simulink model "test"  (R2024b)
settings: Solver=ode4  StartTime=0.0  StopTime=10000  FixedStep=0.01  RelTol=1e-3
values from neighbouring files (symbols this model uses):
  db = 0*[-100 100]    [test_workspace.m]
  dwell_param = [Uon; Uoff; min_on; min_off]    [test_workspace.m]
  Fmax_rcs = 500    [test_workspace.m]
  I = 1e5*diag([1.8382, 1.8626, 1.0379])    [test_workspace.m]
  ka = 0.2*kr    [test_workspace.m]
  km = 4    [test_workspace.m]
  kr = [0.5 0.5 0.8]'    [test_workspace.m]
  larm = 2*[4; 4; 4]    [test_workspace.m]
  min_on = 0.03    [test_workspace.m]
  tau = 1    [test_workspace.m]
  Uoff = 0.1    [test_workspace.m]
  Uon = 0.4    [test_workspace.m]
libraries: simulink x1
settings Model: NumberOfSteps=5000  Creator=gabri  LastModifiedBy=gabri

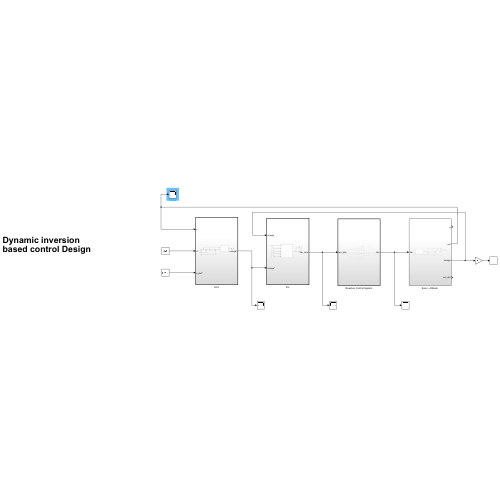
[thumbnail: Simulink's stored preview of the top-level diagram]
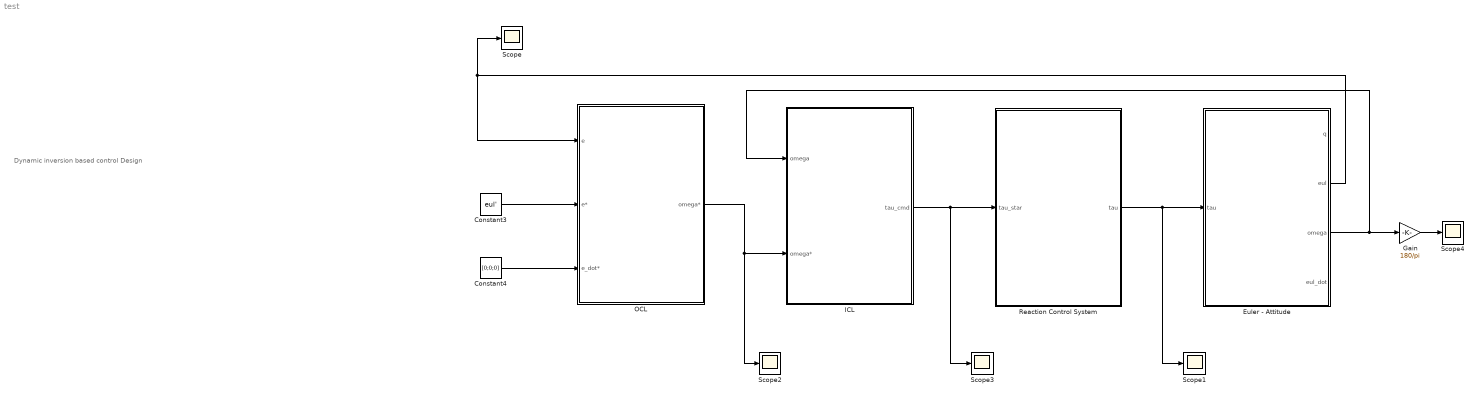
== system test ==
  note: Dynamic inversion based control Design
  Constant3 : Constant  Value=eul'
  Constant4 : Constant  Value=[0;0;0]
  "Euler - Attitude " : Subsystem
  Gain : Gain  Gain=180/pi
  ICL : Subsystem  TreatAsAtomicUnit=on
  OCL : Subsystem  TreatAsAtomicUnit=on
  Reaction Control System : Subsystem  TreatAsAtomicUnit=on
  Scope{,1..4} (5 alike) : Scope
  wires:
  Reaction Control System/1(tau) -> Scope1/1, "Euler - Attitude "/1(tau)
  "Euler - Attitude "/2(eul) -> OCL/1(e), Scope/1
  "Euler - Attitude "/3(omega) -> Gain/1, ICL/1(omega)
  OCL/1(omega*) -> ICL/2(omega*), Scope2/1
  ICL/1(tau_cmd) -> Scope3/1, Reaction Control System/1(tau_star)
  Constant3/1 -> OCL/2(e*)
  Constant4/1 -> OCL/3(e_dot*)
  Gain/1 -> Scope4/1

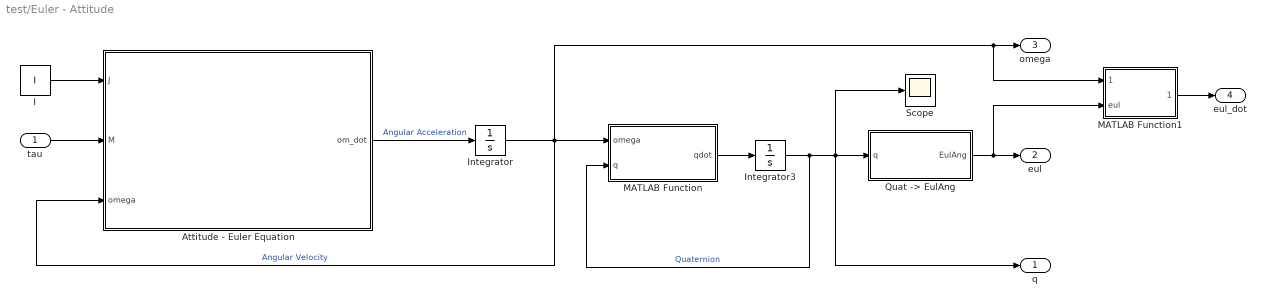
== system test/Euler - Attitude  ==
  tau : Inport
  Attitude - Euler Equation : MATLAB Function  TreatAsAtomicUnit=on
  I : Constant  Value=I
  Integrator : Integrator  InitialCondition=[0; 0; 0]
  Integrator3 : Integrator  InitialCondition=[1; 0; 0; 0]
  MATLAB Function : MATLAB Function  TreatAsAtomicUnit=on
  MATLAB Function1 : MATLAB Function  TreatAsAtomicUnit=on
  "Quat -> EulAng" : MATLAB Function  TreatAsAtomicUnit=on
  Scope : Scope
  q : Outport
  eul : Outport  Port=2
  omega : Outport  Port=3
  eul_dot : Outport  Port=4
  wires:
  Attitude - Euler Equation/1(om_dot) -> Integrator/1  "Angular Acceleration"
  tau/1 -> Attitude - Euler Equation/2(M)
  MATLAB Function/1(qdot) -> Integrator3/1
  Integrator/1 -> MATLAB Function1/1(omega), omega/1, MATLAB Function/1(omega), Attitude - Euler Equation/3(omega)  "Angular Velocity"
  Integrator3/1 -> q/1, "Quat -> EulAng"/1(q), Scope/1, MATLAB Function/2(q)  "Quaternion"
  I/1 -> Attitude - Euler Equation/1(J)
  "Quat -> EulAng"/1(EulAng) -> eul/1, MATLAB Function1/2(eul)
  MATLAB Function1/1(eul_dot) -> eul_dot/1

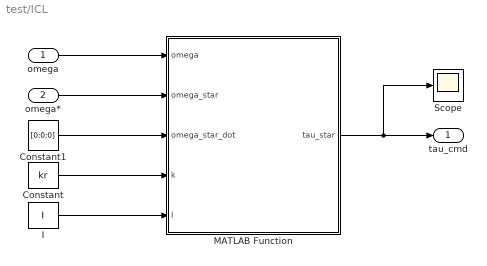
== system test/ICL ==
  omega : Inport
  omega* : Inport  Port=2
  Constant : Constant  Value=kr
  Constant1 : Constant  Value=[0;0;0]
  I : Constant  Value=I
  MATLAB Function : MATLAB Function  TreatAsAtomicUnit=on
  Scope : Scope
  tau_cmd : Outport
  wires:
  omega/1 -> MATLAB Function/1(omega)
  MATLAB Function/1(tau_star) -> Scope/1, tau_cmd/1
  omega*/1 -> MATLAB Function/2(omega_star)
  Constant/1 -> MATLAB Function/4(k)
  I/1 -> MATLAB Function/5(I)
  Constant1/1 -> MATLAB Function/3(omega_star_dot)

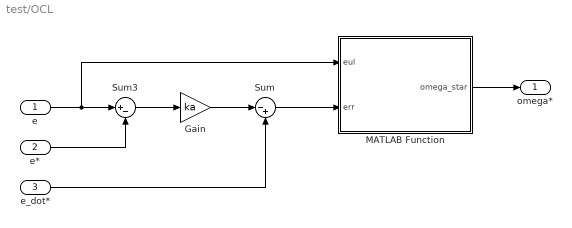
== system test/OCL ==
  e : Inport
  e* : Inport  Port=2
  e_dot* : Inport  Port=3
  Gain : Gain  Gain=ka
  MATLAB Function : MATLAB Function  TreatAsAtomicUnit=on
  Sum : Sum  Inputs=|-+
  Sum3 : Sum  Inputs=|+-
  omega* : Outport
  wires:
  e/1 -> MATLAB Function/1(eul), Sum3/1
  e*/1 -> Sum3/2
  Sum3/1 -> Gain/1
  MATLAB Function/1(omega_star) -> omega*/1
  e_dot*/1 -> Sum/2
  Gain/1 -> Sum/1
  Sum/1 -> MATLAB Function/2(err)

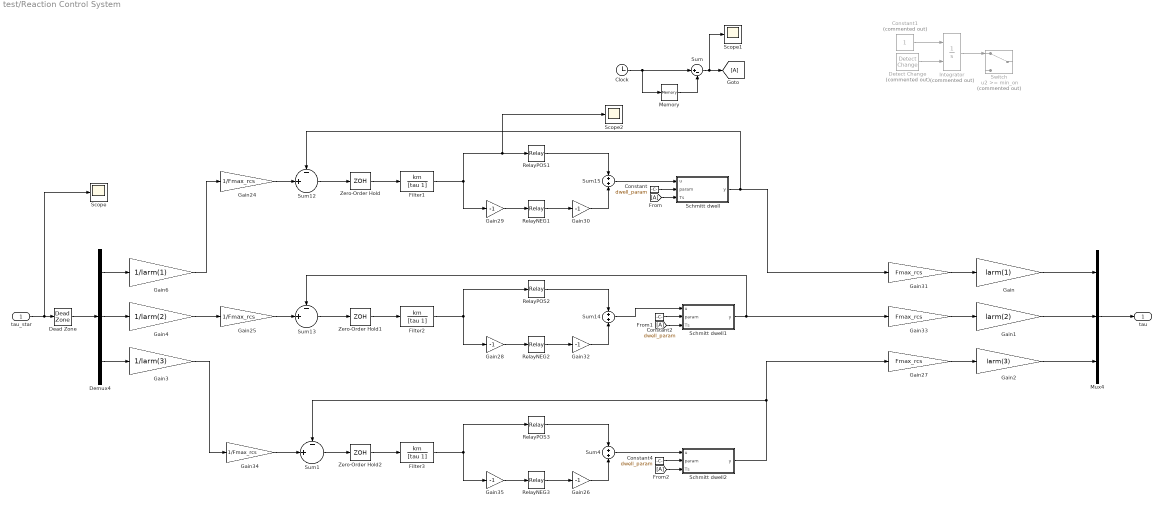
== system test/Reaction Control System ==
  tau_star : Inport
  Clock : Clock
  Constant : Constant  Value=dwell_param
  Constant1 : Constant  Commented=on
  Constant2 : Constant  Value=dwell_param
  Constant4 : Constant  Value=dwell_param
  Dead Zone : DeadZone  LowerValue=db(1)  UpperValue=db(2)
  Demux4 : Demux  Outputs=3
  Detect Change : simulink/Logic and Bit Operations/Detect Change  Commented=on  vinit=0  OutDataTypeStr=boolean
  Filter1 : TransferFcn  Numerator=km  Denominator=[tau 1]
  Filter2 : TransferFcn  Numerator=km  Denominator=[tau 1]
  Filter3 : TransferFcn  Numerator=km  Denominator=[tau 1]
  From : From
  From1 : From
  From2 : From
  Gain : Gain  Gain=larm(1)
  Gain1 : Gain  Gain=larm(2)
  Gain2 : Gain  Gain=larm(3)
  Gain24 : Gain  Gain=1/Fmax_rcs
  Gain25 : Gain  Gain=1/Fmax_rcs
  Gain{26,28..30,32,35} (6 alike) : Gain  Gain=-1
  Gain27 : Gain  Gain=Fmax_rcs
  Gain3 : Gain  Gain=1/larm(3)
  Gain31 : Gain  Gain=Fmax_rcs
  Gain33 : Gain  Gain=Fmax_rcs
  Gain34 : Gain  Gain=1/Fmax_rcs
  Gain4 : Gain  Gain=1/larm(2)
  Gain6 : Gain  Gain=1/larm(1)
  Goto : Goto
  Integrator : Integrator  Commented=on  ExternalReset=level
  Memory : Memory
  Mux4 : Mux  Inputs=3
  RelayNEG1 : Relay  OnSwitchValue=0.45  OffSwitchValue=0.15  ZeroCross=off  SampleTime=0.01
  RelayNEG2 : Relay  OnSwitchValue=Uon  OffSwitchValue=Uoff  ZeroCross=off  SampleTime=0.01
  RelayNEG3 : Relay  OnSwitchValue=0.45  OffSwitchValue=0.15  ZeroCross=off  SampleTime=0.01
  RelayPOS1 : Relay  OnSwitchValue=Uon  OffSwitchValue=Uoff  ZeroCross=off  SampleTime=0.01
  RelayPOS2 : Relay  OnSwitchValue=Uon  OffSwitchValue=Uoff  ZeroCross=off  SampleTime=0.01
  RelayPOS3 : Relay  OnSwitchValue=Uon  OffSwitchValue=Uoff  ZeroCross=off  SampleTime=0.01
  Schmitt dwell : MATLAB Function  TreatAsAtomicUnit=on
  Schmitt dwell1 : MATLAB Function  TreatAsAtomicUnit=on
  Schmitt dwell2 : MATLAB Function  TreatAsAtomicUnit=on
  Scope : Scope
  Scope1 : Scope
  Scope2 : Scope
  Sum : Sum  Inputs=|+-
  Sum1 : Sum  Inputs=-||+|||
  Sum12 : Sum  Inputs=-||+|||
  Sum13 : Sum  Inputs=-||+|||
  Sum14 : Sum  Inputs=+|+
  Sum15 : Sum  Inputs=+|+
  Sum4 : Sum  Inputs=+|+
  Switch : Switch  Commented=on  Threshold=min_on  SaturateOnIntegerOverflow=off  InputSameDT=off
  Zero-Order Hold : ZeroOrderHold  SampleTime=0.01
  Zero-Order Hold1 : ZeroOrderHold  SampleTime=0.01
  Zero-Order Hold2 : ZeroOrderHold  SampleTime=0.01
  tau : Outport
  wires:
  RelayNEG2/1 -> Gain32/1
  RelayNEG3/1 -> Gain26/1
  RelayPOS2/1 -> Sum14/1
  Gain27/1 -> Gain2/1
  Sum4/1 -> Schmitt dwell2/1(u)
  Gain24/1 -> Sum12/2
  Gain30/1 -> Sum15/2
  Filter3/1 -> Gain35/1, RelayPOS3/1
  Gain26/1 -> Sum4/2
  Sum1/1 -> Zero-Order Hold2/1
  Filter2/1 -> Gain28/1, RelayPOS2/1
  RelayPOS3/1 -> Sum4/1
  Demux4/3 -> Gain3/1
  RelayNEG1/1 -> Gain30/1
  Gain28/1 -> RelayNEG2/1
  Demux4/1 -> Gain6/1
  Gain32/1 -> Sum14/2
  Gain31/1 -> Gain/1
  Sum13/1 -> Zero-Order Hold1/1
  Demux4/2 -> Gain4/1
  Sum14/1 -> Schmitt dwell1/1(u)
  Gain33/1 -> Gain1/1
  Gain35/1 -> RelayNEG3/1
  Gain29/1 -> RelayNEG1/1
  Sum12/1 -> Zero-Order Hold/1
  Gain/1 -> Mux4/1
  Gain1/1 -> Mux4/2
  Gain2/1 -> Mux4/3
  tau_star/1 -> Scope/1, Dead Zone/1
  Mux4/1 -> tau/1
  Gain4/1 -> Gain25/1
  Gain3/1 -> Gain34/1
  Integrator/1 -> Switch/1
  Constant1/1 -> Integrator/1
  Detect Change/1 -> Integrator/2
  Sum15/1 -> Schmitt dwell/1(u)
  Filter1/1 -> Scope2/1, RelayPOS1/1, Gain29/1
  RelayPOS1/1 -> Sum15/1
  From/1 -> Schmitt dwell/3(Ts)
  Constant/1 -> Schmitt dwell/2(param)
  Schmitt dwell/1(y) -> Gain31/1, Sum12/1
  Constant2/1 -> Schmitt dwell1/2(param)
  From1/1 -> Schmitt dwell1/3(Ts)
  Schmitt dwell1/1(y) -> Gain33/1, Sum13/1
  Constant4/1 -> Schmitt dwell2/2(param)
  From2/1 -> Schmitt dwell2/3(Ts)
  Schmitt dwell2/1(y) -> Gain27/1, Sum1/1
  Zero-Order Hold/1 -> Filter1/1
  Gain25/1 -> Sum13/2
  Gain34/1 -> Sum1/2
  Zero-Order Hold1/1 -> Filter2/1
  Zero-Order Hold2/1 -> Filter3/1
  Gain6/1 -> Gain24/1
  Dead Zone/1 -> Demux4/1
  Clock/1 -> Memory/1, Sum/1
  Memory/1 -> Sum/2
  Sum/1 -> Scope1/1, Goto/1

== matlab function test/Euler - Attitude /Attitude - Euler Equation ==
  data: J input; om_dot output; M input; omega input
function om_dot = rotation(J, M, omega)
    
    om_dot = inv(J)*(M-cross(omega,J*omega));

end

== matlab function test/Reaction Control System/Schmitt dwell ==
  settings: updateMethod=DISCRETE  sampleTime=0.01
  data: u input; param input; Ts input; y output
function y = schmitt_dwell(u, param, Ts)

    % u: input command (scalar)
    % param = [Uon, Uoff, min_on, min_off]
    % Ts: sample time [s]
    
    persistent state1 ton1 toff1
    
    min_on  = param(3);
    min_off = param(4);
    
    if isempty(state1)
        state1 = 0;   % start OFF
        ton1 = 0; toff1 = 0;
    end
    
    if u>0
        a=1;
    end
    
    % Update timers
    if state1 ~= 0
        ton1  = ton1 + Ts;
        toff1 = 0;
    else
        toff1 = toff1 + Ts;
        ton1  = 0;
    end
    
    if state1 == 0  % currently OFF
        if (u >= 0.5) && (toff1 >= min_off)
            state1 = 1;
            ton1 = 0;
        elseif (u <= -0.5) && (toff1 >= min_off)
            state1 = -1;
            ton1 = 0;
        end
    else  % currently ON (+1 or -1)
        if (abs(u) < 0.5) && (ton1 >= min_on)
            state1 = 0;
            toff1 = 0;
        end
    end
    
    y = state1;

end

== matlab function test/Reaction Control System/Schmitt dwell1 ==
  settings: updateMethod=DISCRETE  sampleTime=0.01
  data: u input; param input; Ts input; y output
function y = schmitt_dwell(u, param, Ts)

    % u: input command (scalar)
    % param = [Uon, Uoff, min_on, min_off]
    % Ts: sample time [s]
    
    persistent state2 ton2 toff2
    
    if u == -1
        a=1;
    end

    min_on  = param(3);
    min_off = param(4);
    
    if isempty(state2)
        state2 = 0;   % start OFF
        ton2 = 0; toff2 = 0;
    end
    
    % Update timers
    if state2 ~= 0
        ton2  = ton2 + Ts;
        toff2 = 0;
    else
        toff2 = toff2 + Ts;
        ton2  = 0;
    end
    
    if state2 == 0  % currently OFF
        if (u >= 0.5) && (toff2 >= min_off)
            state2 = 1;
            ton2 = 0;
        elseif (u <= -0.5) && (toff2 >= min_off)
            state2 = -1;
            ton2 = 0;
        end
    else  % currently ON (+1 or -1)
        if (abs(u) < 0.5) && (ton2 >= min_on)
            state2 = 0;
            toff2 = 0;
        end
    end
    
    y = state2;

end

== matlab function test/Euler - Attitude /MATLAB Function ==
  data: omega input; qdot output; q input
function qdot = fcn(omega,q)

Omega = [0 -omega(1) -omega(2) -omega(3);
         omega(1) 0 omega(3) omega(2);
         omega(2) omega(3) 0 omega(1);
         omega(3) omega(2) omega(1) 0];

q0 = q(1);
q1 = q(2);
q2 = q(3);
q3 = q(4);

qdot = 0.5*Omega*[q0 q1 q2 q3]';

== matlab function test/Euler - Attitude /MATLAB Function1 ==
  data: omega input; eul input; eul_dot output
function eul_dot = fcn(omega, eul)
    
    eul_dot = zeros(3,1);
    eul_dot(1) = omega(1) + omega(2)*sin(eul(1))*tan(eul(2)) + omega(3)*cos(eul(1))*tan(eul(2));
    eul_dot(2) = omega(2)*cos(eul(1)) -  omega(3)*sin(eul(1));
    eul_dot(3) = omega(2)*sin(eul(1))/cos(eul(2)) + omega(3)*cos(eul(1))/cos(eul(2));

end

== matlab function test/Euler - Attitude /Quat -> EulAng ==
  data: q input; EulAng output
function EulAng = fcn(q)

    qs = q(1); qx = q(2); qy = q(3); qz = q(4);
    
    EulAng = [-atan2(2*(-qs*qx+qy*qz), -qx^2-qy^2+qz^2+qs^2);
              atan2(2*(qz*qx+qy*qs), (1-(2*(qz*qx+qy*qs))^2)^.5); %asin(2*(qz*qx+qyqs));
              -atan2(2*(-qs*qz+qx*qy), qx^2-qy^2-qz^2+qs^2)];

end

== matlab function test/ICL/MATLAB Function ==
  data: omega input; tau_star output; omega_star input; omega_star_dot input; k input; I input
function tau_star = fcn(omega, omega_star, omega_star_dot, k ,I)
    
    tau_star = I*(omega_star_dot-k.*(omega-omega_star)) + [(I(3)-I(2))*omega(2)*omega(3); (I(1)-I(3))*omega(1)*omega(3); (I(2)-I(1))*omega(1)*omega(2)];
    % tau_max = 4e3;
    % tau_star = min(max(tau_star, -tau_max), tau_max);

end

== matlab function test/OCL/MATLAB Function ==
  data: eul input; omega_star output; err input
function omega_star = fcn(eul, err)
    
    err = wrapToPi(err);
    T = [1  0 -sin(eul(2));
         0  cos(eul(1)) sin(eul(1))*cos(eul(2));
         0 -sin(eul(1)) cos(eul(1))*cos(eul(2))];
    if err(2)>0
        a=1;
    end
    omega_star = T*err;
    omega_star = max(min(omega_star, 0.7), -0.7);

end

== matlab function test/Reaction Control System/Schmitt dwell2 ==
  settings: updateMethod=DISCRETE  sampleTime=0.01
  data: u input; param input; Ts input; y output
function y = schmitt_dwell(u, param, Ts)

    % u: input command (scalar)
    % param = [Uon, Uoff, min_on, min_off]
    % Ts: sample time [s]
    
    persistent state3 ton3 toff3
    
    if u == -1
        a=1;
    end

    min_on  = param(3);
    min_off = param(4);
    
    if isempty(state3)
        state3 = 0;   % start OFF
        ton3 = 0; toff3 = 0;
    end
    
    % Update timers
    if state3 ~= 0
        ton3  = ton3 + Ts;
        toff3 = 0;
    else
        toff3 = toff3 + Ts;
        ton3  = 0;
    end
    
    if state3 == 0  % currently OFF
        if (u >= 0.5) && (toff3 >= min_off)
            state3 = 1;
            ton3 = 0;
        elseif (u <= -0.5) && (toff3 >= min_off)
            state3 = -1;
            ton3 = 0;
        end
    else  % currently ON (+1 or -1)
        if (abs(u) < 0.5) && (ton3 >= min_on)
            state3 = 0;
            toff3 = 0;
        end
    end
    
    y = state3;

end
